simulink model "EOM"  (R2015b)
settings: Solver=VariableStepAuto  StartTime=0.0  StopTime=10.0  RelTol=1e-3
libraries: aerolib6dof2 x1
settings Model: Creator=Pramod  LastModifiedBy=Pramod

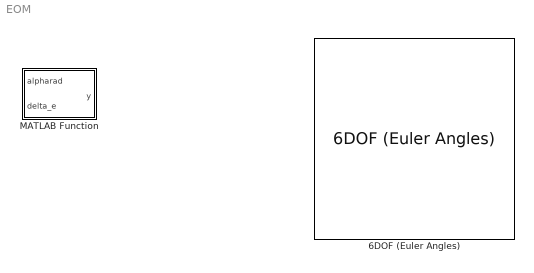
== system EOM ==
  6DOF (Euler Angles) : aerolib6dof2/6DOF (Euler Angles)  units=Metric (MKS)  mtype=Fixed  rep=Euler Angles  xme_0=[0 0 0]  Vm_0=[0 0 0]  eul_0=[0 0 0]  pm_0=[0 0 0]  mass_0=1.0  mass_e=0.5  mass_f=2.0  inertia=eye(3)  inertia_e=eye(3)  inertia_f=2*eye(3)  k_quat=1.0  vre_flag=on
  MATLAB Function : MATLAB Function  TreatAsAtomicUnit=on

== matlab function EOM/MATLAB Function ==
  data: alpharad input; y output; delta_e input
function y = fcn(alpharad,delta_e)
F_X=y(1);
F_Z=y(2);
M=y(3);
g = 9.8;
rho = 1.225;
m = 1043.26;
C_bar = 1.493;
b = 10.911;
S_ref = 16.1651;
delta_e= -0.1383;
T=1.2109e+04;
C_L_0 = 0.25;
C_L_alpha = 4.47;
C_L_q = 1.7;
C_L_delta_e = 0.3476;
C_D_0 = 0.036;
k = 0.3;
C_M_0 = -0.02;
C_M_alpha = -1.8;
C_M_alpha_dot = -12.4;
C_M_delta_e = -1.28;
C_L = C_L_0 + C_L_alpha*alpharad +   C_L_delta_e*delta_e;
C_D = C_D_0 + k*C_L^2;
C_M = C_M_0 + C_M_alpha*alpharad +  C_M_delta_e*delta_e;
C_X = -C_D*cos(alpharad) + C_L*sin(alpharad);
C_Z = -C_D*sin(alpharad) - C_L*cos(alpharad);
F_X=0.5*rho*V^2*S_ref*C_X;
F_Z=0.5*rho*V^2*S_ref*C_Z;
M=rho*V^2*S_ref*C_bar*C_M
